simulink model "SHE"  (R2016b)
settings: Solver=VariableStepAuto  StartTime=0.0  StopTime=0.06  RelTol=1e-3
libraries: powerlib x31
settings Model: Creator=Youssef  LastModifiedBy=Youssef

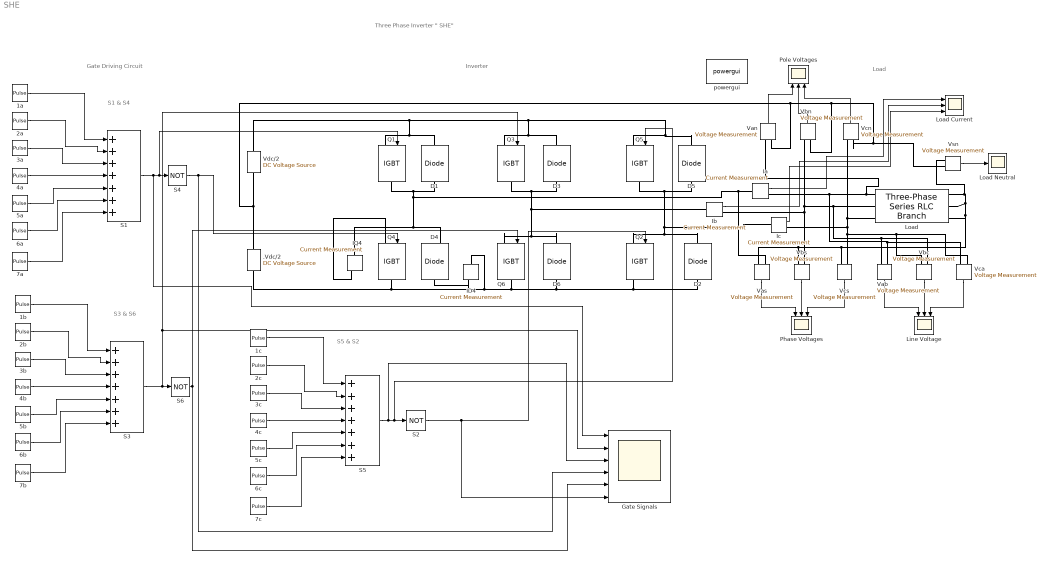
== system SHE ==
  note: Gate Driving Circuit
  note: Load
  note: Inverter
  note: S1 & S4
  note: S3 & S6
  note: Three Phase Inverter " SHE"
  note: S5 & S2
  .Vdc/2 : powerlib/Electrical Sources/DC Voltage Source  Amplitude=100  Measurements=None
  1a : DiscretePulseGenerator  PulseType=Time based  Period=0.02  PulseWidth=(0.5937-0.2076)*100/(2*pi)  PhaseDelay=0.0007
  1b : DiscretePulseGenerator  PulseType=Time based  Period=0.02  PulseWidth=(0.5937-0.2076)*100/(2*pi)  PhaseDelay=0.0007+(0.02/3)
  1c : DiscretePulseGenerator  PulseType=Time based  Period=0.02  PulseWidth=(0.5937-0.2076)*100/(2*pi)  PhaseDelay=0.0007+(2*0.02/3)
  2a : DiscretePulseGenerator  PulseType=Time based  Period=0.02  PulseWidth=(pi-2*0.6523)*100/(2*pi)  PhaseDelay=0.0021
  2b : DiscretePulseGenerator  PulseType=Time based  Period=0.02  PulseWidth=(pi-2*0.6523)*100/(2*pi)  PhaseDelay=0.0021+(0.02/3)
  2c : DiscretePulseGenerator  PulseType=Time based  Period=0.02  PulseWidth=(pi-2*0.6523)*100/(2*pi)  PhaseDelay=0.0021+(2*0.02/3)
  3a : DiscretePulseGenerator  PulseType=Time based  Period=0.02  PulseWidth=(0.5937-0.2076)*100/(2*pi)  PhaseDelay=(pi-0.5937)*0.02/(2*pi)
  3b : DiscretePulseGenerator  PulseType=Time based  Period=0.02  PulseWidth=(0.5937-0.2076)*100/(2*pi)  PhaseDelay=(pi-0.5937)*0.02/(2*pi)+(0.02/3)
  3c : DiscretePulseGenerator  PulseType=Time based  Period=0.02  PulseWidth=(0.5937-0.2076)*100/(2*pi)  PhaseDelay=(pi-0.5937)*0.02/(2*pi)+(2*0.02/3)
  4a : DiscretePulseGenerator  PulseType=Time based  Period=0.02  PulseWidth=0.2076*100/(2*pi)  PhaseDelay=0.02/2
  4b : DiscretePulseGenerator  PulseType=Time based  Period=0.02  PulseWidth=0.2076*100/(2*pi)  PhaseDelay=0.02/2+(0.02/3)
  4c : DiscretePulseGenerator  PulseType=Time based  Period=0.02  PulseWidth=0.2076*100/(2*pi)  PhaseDelay=0.02/2+(2*0.02/3)
  5a : DiscretePulseGenerator  PulseType=Time based  Period=0.02  PulseWidth=(0.6523-0.5937)*100/(2*pi)  PhaseDelay=(pi+0.5937)*0.02/(2*pi)
  5b : DiscretePulseGenerator  PulseType=Time based  Period=0.02  PulseWidth=(0.6523-0.5937)*100/(2*pi)  PhaseDelay=(pi+0.5937)*0.02/(2*pi)+(0.02/3)
  5c : DiscretePulseGenerator  PulseType=Time based  Period=0.02  PulseWidth=(0.6523-0.5937)*100/(2*pi)  PhaseDelay=(pi+0.5937)*0.02/(2*pi)+(2*0.02/3)
  6a : DiscretePulseGenerator  PulseType=Time based  Period=0.02  PulseWidth=(0.6523-0.5937)*100/(2*pi)  PhaseDelay=(2*pi-0.6523)*0.02/(2*pi)
  6b : DiscretePulseGenerator  PulseType=Time based  Period=0.02  PulseWidth=(0.6523-0.5937)*100/(2*pi)  PhaseDelay=(2*pi-0.6523)*0.02/(2*pi)+(0.02/3)
  6c : DiscretePulseGenerator  PulseType=Time based  Period=0.02  PulseWidth=(0.6523-0.5937)*100/(2*pi)  PhaseDelay=(2*pi-0.6523)*0.02/(2*pi)+(2*0.02/3)
  7a : DiscretePulseGenerator  PulseType=Time based  Period=0.02  PulseWidth=0.2076*100/(2*pi)  PhaseDelay=((2*pi)-0.2076)*0.02/(2*pi)
  7b : DiscretePulseGenerator  PulseType=Time based  Period=0.02  PulseWidth=0.2076*100/(2*pi)  PhaseDelay=((2*pi)-0.2076)*0.02/(2*pi)+(0.02/3)
  7c : DiscretePulseGenerator  PulseType=Time based  Period=0.02  PulseWidth=0.2076*100/(2*pi)  PhaseDelay=((2*pi)-0.2076)*0.02/(2*pi)+(2*0.02/3)
  D{1..3,5..6} (5 alike) : powerlib/Power Electronics/Diode  Ron=0.001  Lon=0  Vf=0.8  IC=0  UseSnubber=off  Rs=500  Cs=250e-9  Measurements=off
  D4 : powerlib/Power Electronics/Diode  Ron=0.001  Lon=0  Vf=0.8  IC=0  UseSnubber=off  Rs=500  Cs=250e-9  Measurements=on
  Gate Signals : Scope  NumInputPorts=6
  ID4 : powerlib/Measurements/Current Measurement  PhasorSimulation=off  OutputType=Complex  PSBequivalent=0
  IQ4 : powerlib/Measurements/Current Measurement  PhasorSimulation=off  OutputType=Complex  PSBequivalent=0
  Ia : powerlib/Measurements/Current Measurement  PhasorSimulation=off  OutputType=Complex  PSBequivalent=0
  Ib : powerlib/Measurements/Current Measurement  PhasorSimulation=off  OutputType=Complex  PSBequivalent=0
  Ic : powerlib/Measurements/Current Measurement  PhasorSimulation=off  OutputType=Complex  PSBequivalent=0
  Line Voltage : Scope  NumInputPorts=3
  Load : powerlib/Elements/Three-Phase Series RLC Branch  LConnTagsString=A|B|C  RConnTagsString=A|B|C  BranchType=R  Resistance=1  Inductance=1e-3  Capacitance=1e-6  Measurements=None
  Load Current : Scope  NumInputPorts=3
  Load Neutral : Scope
  Phase Voltages : Scope  NumInputPorts=3
  Pole Voltages : Scope  NumInputPorts=3
  Q{1,3..6} (5 alike) : powerlib/Power Electronics/IGBT  Ron=0.001  Lon=0  Vf=0.4  Tf=1e-6  Tt=2e-6  IC=0  Rs=1e5  Cs=inf  Measurements=off
  Q2 : powerlib/Power Electronics/IGBT  Ron=0.001  Lon=0  Vf=0.4  Tf=1e-6  Tt=2e-6  IC=0  Rs=1e5  Cs=inf  Measurements=on
  S1 : Sum  Inputs=7
  S2 : Logic  Operator=NOT  AllPortsSameDT=off  OutDataTypeStr=boolean
  S3 : Sum  Inputs=7
  S4 : Logic  Operator=NOT  AllPortsSameDT=off  OutDataTypeStr=boolean
  S5 : Sum  Inputs=7
  S6 : Logic  Operator=NOT  AllPortsSameDT=off  OutDataTypeStr=boolean
  Vab : powerlib/Measurements/Voltage Measurement  PhasorSimulation=off  OutputType=Complex  PSBequivalent=0
  Van : powerlib/Measurements/Voltage Measurement  PhasorSimulation=off  OutputType=Complex  PSBequivalent=0
  Vas : powerlib/Measurements/Voltage Measurement  PhasorSimulation=off  OutputType=Complex  PSBequivalent=0
  Vbc : powerlib/Measurements/Voltage Measurement  PhasorSimulation=off  OutputType=Complex  PSBequivalent=0
  Vbn : powerlib/Measurements/Voltage Measurement  PhasorSimulation=off  OutputType=Complex  PSBequivalent=0
  Vbs : powerlib/Measurements/Voltage Measurement  PhasorSimulation=off  OutputType=Complex  PSBequivalent=0
  Vca : powerlib/Measurements/Voltage Measurement  PhasorSimulation=off  OutputType=Complex  PSBequivalent=0
  Vcn : powerlib/Measurements/Voltage Measurement  PhasorSimulation=off  OutputType=Complex  PSBequivalent=0
  Vcs : powerlib/Measurements/Voltage Measurement  PhasorSimulation=off  OutputType=Complex  PSBequivalent=0
  Vdc/2 : powerlib/Electrical Sources/DC Voltage Source  Amplitude=100  Measurements=None
  Vsn : powerlib/Measurements/Voltage Measurement  PhasorSimulation=off  OutputType=Complex  PSBequivalent=0
  powergui : powerlib/powergui  Priority=1  SimulationMode=Discrete  SolverType=Tustin/Backward Euler (TBE)  SampleTime=1e-6  frequency=60  SPID=off  DisableSnubberDevices=off  DisableRonSwitches=off  DisableVfSwitches=off  SwTol=0  DisplayEquations=off  Interpol=off  ExternalGateDelay=off  methode=off  Ts=10  FunctionMessages=off  echomessages=off  HookPort=off  EnableUseOfTLC=off  x0status=blocks  frequencyindice=0  Pbase=100e6  ErrMax=1e-4  Iterations=50  UnitsV=kV  UnitsW=MW  buscounter=0  RestoreLinks=warning  ResistiveCurrentMeasurement=off  Frange=[0:2:500]  Ylog=off  Xlog=on  ShowGrid=off  save=off  variable=ZData  structure=V  ZoomFFT=on  StartTime=0.02  cycles=2  DisplayStyle=1  fundamental=50  FreqAxis=off  MaxFrequency=1000  frequencyindicesteady=1  RmsSteady=1  display=off
  wires:
  Ia/1 -> Load Current/1
  Ib/1 -> Load Current/2
  Ic/1 -> Load Current/3
  Van/1 -> Pole Voltages/1
  Vbn/1 -> Pole Voltages/2
  Vcn/1 -> Pole Voltages/3
  Vas/1 -> Phase Voltages/1
  Vbs/1 -> Phase Voltages/2
  Vcs/1 -> Phase Voltages/3
  Vab/1 -> Line Voltage/1
  Vbc/1 -> Line Voltage/2
  Vca/1 -> Line Voltage/3
  Vsn/1 -> Load Neutral/1
  1a/1 -> S1/1
  2a/1 -> S1/2
  3a/1 -> S1/3
  4a/1 -> S1/4
  5a/1 -> S1/5
  6a/1 -> S1/6
  7a/1 -> S1/7
  S1/1 -> Gate Signals/1, Q1/1, S4/1
  1b/1 -> S3/1
  2b/1 -> S3/2
  3b/1 -> S3/3
  4b/1 -> S3/4
  5b/1 -> S3/5
  6b/1 -> S3/6
  7b/1 -> S3/7
  S3/1 -> Q3/1, Gate Signals/2, S6/1
  1c/1 -> S5/1
  2c/1 -> S5/2
  3c/1 -> S5/3
  4c/1 -> S5/4
  5c/1 -> S5/5
  6c/1 -> S5/6
  7c/1 -> S5/7
  S5/1 -> Gate Signals/3, Q5/1, S2/1
  S4/1 -> Gate Signals/4, Q4/1
  S6/1 -> Q6/1, Gate Signals/5
  S2/1 -> Gate Signals/6, Q2/1
  connections:
  Vdc/2/RConn1 -- D5/RConn1 -- Q5/LConn1 -- Q3/LConn1 -- D3/RConn1 -- Q1/LConn1 -- D1/RConn1
  Q6/LConn1 -- D6/RConn1 -- Ib/LConn1 -- D3/LConn1 -- Q3/RConn1
  Ic/LConn1 -- D2/RConn1 -- Q2/LConn1 -- Q5/RConn1 -- D5/LConn1
  Van/LConn2 -- Vsn/LConn2 -- Vcn/LConn2 -- Vbn/LConn2 -- .Vdc/2/RConn1 -- Vdc/2/LConn1
  .Vdc/2/LConn1 -- Q4/RConn1 -- ID4/LConn1 -- D2/LConn1 -- Q2/RConn1 -- D6/LConn1 -- Q6/RConn1
  Vsn/LConn1 -- Load/RConn1 -- Load/RConn2 -- Vas/LConn2 -- Vbs/LConn2 -- Vcs/LConn2 -- Load/RConn3
  Vab/LConn1 -- Vca/LConn2 -- Ia/RConn1 -- Load/LConn1 -- Van/LConn1
  Vbn/LConn1 -- Vab/LConn2 -- Vbc/LConn1 -- Load/LConn2 -- Vbs/LConn1 -- Ib/RConn1
  Vcs/LConn1 -- Vca/LConn1 -- Vbc/LConn2 -- Ic/RConn1 -- Load/LConn3 -- Vcn/LConn1
  IQ4/LConn1 -- D4/RConn1 -- Vas/LConn1 -- Ia/LConn1 -- Q1/RConn1 -- D1/LConn1
  ID4/RConn1 -- D4/LConn1
  IQ4/RConn1 -- Q4/LConn1
